simulink model "distributed_project_triangle_adjusted"  (R2025b)
settings: Solver=VariableStepAuto  StartTime=0.0  StopTime=10  RelTol=1e-3  AbsTol=1e-3  EnableMultiTasking=on
model workspace (MAT data in the model file):
  t_now = 10
  v = 1
values from neighbouring files (symbols this model uses):
  m = 20    [FirstRegression.m]
  msg_init =     [distributed_project_adjusted.mat]
  N = min([length(e1), length(e2), length(e3), N_max])    [10_runs_result_for_odometer.m]    (also in cc.m = min(length(e1), length(e2)); distributed_project_adjusted.mat = 100; distributed_stats.m = min([length(e1),length(e2),length(e3)]); ten_runs_result_for_odometer.m)
  r = 0.05    [distributed_project.mat]    (also in distributed_project_adjusted.mat)
undefined symbols (not defined in the file or in its folder): fractalcoef, X, Y, Z
libraries: nesl_utility x52, sm_lib x38, simulink x15, matrix_library x15, mspfiltlib x3, sensorgpslib x3, mspsensorlib x3
(part 3 of 4)

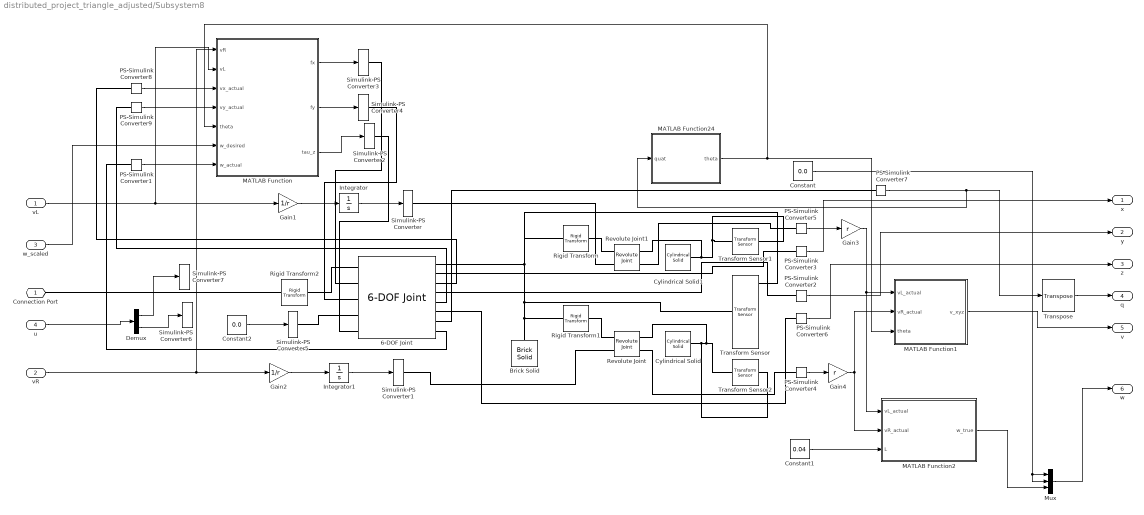
== system distributed_project_triangle_adjusted/Subsystem8 ==
  vL : Inport  PortDimensions=1  SampleTime=0.01
  vR : Inport  Port=2  PortDimensions=1  SampleTime=0.01
  w_scaled : Inport  Port=3
  u : Inport  Port=4  PortDimensions=[2 1]  SampleTime=0.01
  6-DOF Joint : sm_lib/Joints/6-DOF Joint  JointMode=Normal  CompositeWrenchDir=FollowerOnBase  CompositeWrenchFrame=BaseFrame  SenseConstraintForce=off  SenseConstraintTorque=off  SenseTotalForce=off  SenseTotalTorque=off  PxPositionTargetSpecify=on  PxPositionTargetPriority=High  PxPositionTargetValue=0  PxPositionTargetValueUnits=m  PxVelocityTargetSpecify=off  PxVelocityTargetPriority=High  PxVelocityTargetValue=0  PxVelocityTargetValueUnits=m/s  PxEquilibriumPosition=0  PxEquilibriumPositionUnits=m  PxSpringStiffness=0  PxSpringStiffnessUnits=N/m  PxDampingCoefficient=0  PxDampingCoefficientUnits=N/(m/s)  PxLowerLimitSpecify=off  PxLowerLimitBound=-1  PxLowerLimitBoundUnits=m  PxLowerLimitStiffness=1e6  PxLowerLimitStiffnessUnits=N/m  PxLowerLimitDamping=1e3  PxLowerLimitDampingUnits=N/(m/s)  PxLowerLimitTransitionRegionWidth=1e-4  PxLowerLimitTransitionRegionWidthUnits=m  PxUpperLimitSpecify=off  PxUpperLimitBound=1  PxUpperLimitBoundUnits=m  PxUpperLimitStiffness=1e6  PxUpperLimitStiffnessUnits=N/m  PxUpperLimitDamping=1e3  PxUpperLimitDampingUnits=N/(m/s)  PxUpperLimitTransitionRegionWidth=1e-4  PxUpperLimitTransitionRegionWidthUnits=m  PxTorqueActuationMode=InputTorque  PxMotionActuationMode=ComputedMotion  PxSensePosition=on  PxSenseVelocity=on  PxSenseAcceleration=off  PxSenseTorqueForce=off  PxSenseLowerLimitTorqueForce=off  PxSenseUpperLimitTorqueForce=off  PyPositionTargetSpecify=on  PyPositionTargetPriority=High  PyPositionTargetValue=0  PyPositionTargetValueUnits=m  PyVelocityTargetSpecify=off  PyVelocityTargetPriority=High  PyVelocityTargetValue=0  PyVelocityTargetValueUnits=m/s  PyEquilibriumPosition=0  PyEquilibriumPositionUnits=m  PySpringStiffness=0  PySpringStiffnessUnits=N/m  PyDampingCoefficient=0  PyDampingCoefficientUnits=N/(m/s)  PyLowerLimitSpecify=off  PyLowerLimitBound=-1  PyLowerLimitBoundUnits=m  PyLowerLimitStiffness=1e6  PyLowerLimitStiffnessUnits=N/m  PyLowerLimitDamping=1e3  PyLowerLimitDampingUnits=N/(m/s)  PyLowerLimitTransitionRegionWidth=1e-4  PyLowerLimitTransitionRegionWidthUnits=m  PyUpperLimitSpecify=off  PyUpperLimitBound=1  PyUpperLimitBoundUnits=m  PyUpperLimitStiffness=1e6  PyUpperLimitStiffnessUnits=N/m  PyUpperLimitDamping=1e3  PyUpperLimitDampingUnits=N/(m/s)  PyUpperLimitTransitionRegionWidth=1e-4  PyUpperLimitTransitionRegionWidthUnits=m  PyTorqueActuationMode=InputTorque  PyMotionActuationMode=ComputedMotion  PySensePosition=on  PySenseVelocity=on  PySenseAcceleration=off  PySenseTorqueForce=off  PySenseLowerLimitTorqueForce=off  PySenseUpperLimitTorqueForce=off  PzPositionTargetSpecify=on  PzPositionTargetPriority=High  PzPositionTargetValue=0.075  PzPositionTargetValueUnits=m  PzVelocityTargetSpecify=on  PzVelocityTargetPriority=High  PzVelocityTargetValue=0  PzVelocityTargetValueUnits=m/s  PzEquilibriumPosition=0  PzEquilibriumPositionUnits=m  PzSpringStiffness=0  PzSpringStiffnessUnits=N/m  PzDampingCoefficient=0  PzDampingCoefficientUnits=N/(m/s)  PzLowerLimitSpecify=off  PzLowerLimitBound=-1  PzLowerLimitBoundUnits=m  PzLowerLimitStiffness=1e6  PzLowerLimitStiffnessUnits=N/m  PzLowerLimitDamping=1e3  PzLowerLimitDampingUnits=N/(m/s)  PzLowerLimitTransitionRegionWidth=1e-4  PzLowerLimitTransitionRegionWidthUnits=m  PzUpperLimitSpecify=off  PzUpperLimitBound=1  PzUpperLimitBoundUnits=m  PzUpperLimitStiffness=1e6  PzUpperLimitStiffnessUnits=N/m  PzUpperLimitDamping=1e3  PzUpperLimitDampingUnits=N/(m/s)  PzUpperLimitTransitionRegionWidth=1e-4  PzUpperLimitTransitionRegionWidthUnits=m  PzTorqueActuationMode=ComputedTorque  PzMotionActuationMode=InputMotion  PzSensePosition=on  PzSenseVelocity=off  PzSenseAcceleration=off  PzSenseTorqueForce=off  PzSenseLowerLimitTorqueForce=off  PzSenseUpperLimitTorqueForce=off  SphPositionTargetSpecify=on  SphPositionTargetPriority=High  SphPositionTargetRotationMethod=StandardAxis  SphPositionTargetFollAlignAxisA=+X  SphPositionTargetBaseAlignAxisA=+Y  SphPositionTargetFollAlignAxisB=+Y  SphPositionTargetBaseAlignAxisB=+Z  SphPositionTargetRotationStandardAxis=+Z  SphPositionTargetRotationAngle=0.0  SphPositionTargetRotationAngleUnits=rad  SphPositionTargetRotationArbitraryAxis=[0 0 1]  SphPositionTargetRotationSequenceAxes=FollowerAxes  SphPositionTargetRotationSequence=XYX  SphPositionTargetRotationSequenceAngles=[0 0 0]  SphPositionTargetRotationSequenceAnglesUnits=deg  SphPositionTargetRotationMatrix=[1 0 0;0 1 0;0 0 1]  SphPositionTargetQuaternion=[1 0 0 0]  SphVelocityTargetSpecify=off  SphVelocityTargetPriority=High  SphVelocityTargetValue=[0 0 0]  SphVelocityTargetValueUnits=rad/s  SphVelocityTargetInFollowerFrame=on  SphEqPosRotationMethod=None  SphEqPosFollAlignAxisA=+X  SphEqPosBaseAlignAxisA=+Y  SphEqPosFollAlignAxisB=+Y  SphEqPosBaseAlignAxisB=+Z  SphEqPosRotationStandardAxis=+Z  SphEqPosRotationAngle=0  SphEqPosRotationAngleUnits=deg  SphEqPosRotationArbitraryAxis=[0 0 1]  SphEqPosRotationSequenceAxes=FollowerAxes  SphEqPosRotationSequence=XYX  SphEqPosRotationSequenceAngles=[0 0 0]  SphEqPosRotationSequenceAnglesUnits=deg  SphEqPosRotationMatrix=[1 0 0;0 1 0;0 0 1]  SphEqPosQuaternion=[1 0 0 0]  SphSpringStiffness=0  SphSpringStiffnessUnits=N*m/deg  SphDampingCoefficient=0  SphDampingCoefficientUnits=N*m/(deg/s)  SphLowerLimitSpecify=off  SphLowerLimitBound=15  SphLowerLimitBoundUnits=deg  SphLowerLimitStiffness=1e4  SphLowerLimitStiffnessUnits=N*m/deg  SphLowerLimitDamping=10  SphLowerLimitDampingUnits=N*m/(deg/s)  SphLowerLimitTransitionRegionWidth=0.1  SphLowerLimitTransitionRegionWidthUnits=deg  SphUpperLimitSpecify=off  SphUpperLimitBound=45  SphUpperLimitBoundUnits=deg  SphUpperLimitStiffness=1e4  SphUpperLimitStiffnessUnits=N*m/deg  SphUpperLimitDamping=10  SphUpperLimitDampingUnits=N*m/(deg/s)  SphUpperLimitTransitionRegionWidth=0.1  SphUpperLimitTransitionRegionWidthUnits=deg  SphTorqueActuationMode=InputTorque  SphActuateTorqueX=off  SphActuateTorqueY=off  SphActuateTorqueZ=on  SphActuateTorque=off  SphActuationFrame=BaseFrame  SphSensePosition=on  SphSenseVelocityX=off  SphSenseVelocityY=off  SphSenseVelocityZ=on  SphSenseVelocity=off  SphSenseAccelerationX=off  SphSenseAccelerationY=off  SphSenseAccelerationZ=off  SphSenseAcceleration=off  SphSenseLowerLimitTorqueMag=off  SphSenseUpperLimitTorqueMag=off  SphSensingFrame=BaseFrame
  Brick Solid : sm_lib/Body Elements/Brick Solid  BrickDimensions=[0.3 0.15 0.2]  BrickDimensionsUnits=m  ExportEntireGeometry=off  InertiaType=CalculateFromGeometry  BasedOnType=Density  Density=1000  DensityUnits=kg/m^3  Mass=1  MassUnits=kg  CenterOfMass=[0 0 0]  CenterOfMassUnits=m  MomentsOfInertia=[1 1 1]  MomentsOfInertiaUnits=kg*m^2  ProductsOfInertia=[0 0 0]  ProductsOfInertiaUnits=kg*m^2  GraphicType=FromGeometry  MarkerShape=Sphere  MarkerSize=10  GraphicVisPropType=AdvancedVisualProperties  GraphicDiffuseColor=[0.5 0.5 0.5]  GraphicOpacity=1.0  GraphicSpecularColor=[0.5 0.5 0.5 1.0]  GraphicAmbientColor=[0.15 0.15 0.15 1.0]  GraphicEmissiveColor=[0.0 0.0 0.0 1.0]  GraphicShininess=75  DoExposeReferenceFrame=on  SerializedFrames=<Frames/>
  Constant : Constant  Value=0.0  SampleTime=0.01
  Constant1 : Constant  Value=0.04  SampleTime=0.01
  Constant2 : Constant  Value=0.0  SampleTime=0.01
  Cylindrical Solid : sm_lib/Body Elements/Cylindrical Solid  CylinderRadius=0.05  CylinderRadiusUnits=m  CylinderLength=0.04  CylinderLengthUnits=m  ExportEntireGeometry=off  InertiaType=CalculateFromGeometry  BasedOnType=Density  Density=1000  DensityUnits=kg/m^3  Mass=1  MassUnits=kg  CenterOfMass=[0 0 0]  CenterOfMassUnits=m  MomentsOfInertia=[1 1 1]  MomentsOfInertiaUnits=kg*m^2  ProductsOfInertia=[0 0 0]  ProductsOfInertiaUnits=kg*m^2  GraphicType=FromGeometry  MarkerShape=Sphere  MarkerSize=10  GraphicVisPropType=SimpleVisualProperties  GraphicDiffuseColor=[0.5 0.5 0.5]  GraphicOpacity=1  GraphicSpecularColor=[0.5 0.5 0.5 1.0]  GraphicAmbientColor=[0.15 0.15 0.15 1.0]  GraphicEmissiveColor=[0.0 0.0 0.0 1.0]  GraphicShininess=75  DoExposeReferenceFrame=on  SerializedFrames=<Frames/>
  Cylindrical Solid1 : sm_lib/Body Elements/Cylindrical Solid  CylinderRadius=0.05  CylinderRadiusUnits=m  CylinderLength=0.04  CylinderLengthUnits=m  ExportEntireGeometry=off  InertiaType=CalculateFromGeometry  BasedOnType=Density  Density=1000  DensityUnits=kg/m^3  Mass=1  MassUnits=kg  CenterOfMass=[0 0 0]  CenterOfMassUnits=m  MomentsOfInertia=[1 1 1]  MomentsOfInertiaUnits=kg*m^2  ProductsOfInertia=[0 0 0]  ProductsOfInertiaUnits=kg*m^2  GraphicType=FromGeometry  MarkerShape=Sphere  MarkerSize=10  GraphicVisPropType=SimpleVisualProperties  GraphicDiffuseColor=[0.5 0.5 0.5]  GraphicOpacity=1  GraphicSpecularColor=[0.5 0.5 0.5 1.0]  GraphicAmbientColor=[0.15 0.15 0.15 1.0]  GraphicEmissiveColor=[0.0 0.0 0.0 1.0]  GraphicShininess=75  DoExposeReferenceFrame=on  SerializedFrames=<Frames/>
  Demux : Demux  Outputs=2
  Gain1 : Gain  Gain=1/r
  Gain2 : Gain  Gain=1/r
  Gain3 : Gain  Gain=r
  Gain4 : Gain  Gain=r
  Integrator : Integrator
  Integrator1 : Integrator
  MATLAB Function : MATLAB Function  TreatAsAtomicUnit=on
  MATLAB Function1 : MATLAB Function  TreatAsAtomicUnit=on
  MATLAB Function2 : MATLAB Function  TreatAsAtomicUnit=on
  MATLAB Function24 : MATLAB Function  TreatAsAtomicUnit=on
  Mux : Mux  Inputs=3
  PS-Simulink Converter{1..9} (9 alike) : nesl_utility/PS-Simulink Converter  PhysicalDomain=network_engine_domain  SubClassName=ps_output  LeftPortType=input  RightPortType=output  PseudoPeriodic=off  Frequencies=[]  VectorFormat=inherit  Unit=inherit  AffineConversion=off
  Revolute Joint : sm_lib/Joints/Revolute Joint  JointMode=Normal  CompositeWrenchDir=FollowerOnBase  CompositeWrenchFrame=BaseFrame  SenseConstraintForce=off  SenseConstraintTorque=off  SenseTotalForce=off  SenseTotalTorque=off  PositionTargetSpecify=off  PositionTargetPriority=High  PositionTargetValue=0  PositionTargetValueUnits=rad  VelocityTargetSpecify=off  VelocityTargetPriority=High  VelocityTargetValue=0  VelocityTargetValueUnits=rad/s  EquilibriumPosition=0  EquilibriumPositionUnits=deg  SpringStiffness=0  SpringStiffnessUnits=N*m/deg  DampingCoefficient=0  DampingCoefficientUnits=N*m/(deg/s)  LowerLimitSpecify=off  LowerLimitBound=-90  LowerLimitBoundUnits=deg  LowerLimitStiffness=1e4  LowerLimitStiffnessUnits=N*m/deg  LowerLimitDamping=10  LowerLimitDampingUnits=N*m/(deg/s)  LowerLimitTransitionRegionWidth=0.1  LowerLimitTransitionRegionWidthUnits=deg  UpperLimitSpecify=off  UpperLimitBound=90  UpperLimitBoundUnits=deg  UpperLimitStiffness=1e4  UpperLimitStiffnessUnits=N*m/deg  UpperLimitDamping=10  UpperLimitDampingUnits=N*m/(deg/s)  UpperLimitTransitionRegionWidth=0.1  UpperLimitTransitionRegionWidthUnits=deg  TorqueActuationMode=ComputedTorque  MotionActuationMode=InputMotion  SensePosition=off  SenseVelocity=on  SenseAcceleration=off  SenseTorqueForce=off  SenseLowerLimitTorqueForce=off  SenseUpperLimitTorqueForce=off
  Revolute Joint1 : sm_lib/Joints/Revolute Joint  JointMode=Normal  CompositeWrenchDir=FollowerOnBase  CompositeWrenchFrame=BaseFrame  SenseConstraintForce=off  SenseConstraintTorque=off  SenseTotalForce=off  SenseTotalTorque=off  PositionTargetSpecify=off  PositionTargetPriority=High  PositionTargetValue=0  PositionTargetValueUnits=rad  VelocityTargetSpecify=off  VelocityTargetPriority=High  VelocityTargetValue=0  VelocityTargetValueUnits=rad/s  EquilibriumPosition=0  EquilibriumPositionUnits=deg  SpringStiffness=0  SpringStiffnessUnits=N*m/deg  DampingCoefficient=0  DampingCoefficientUnits=N*m/(deg/s)  LowerLimitSpecify=off  LowerLimitBound=-90  LowerLimitBoundUnits=deg  LowerLimitStiffness=1e4  LowerLimitStiffnessUnits=N*m/deg  LowerLimitDamping=10  LowerLimitDampingUnits=N*m/(deg/s)  LowerLimitTransitionRegionWidth=0.1  LowerLimitTransitionRegionWidthUnits=deg  UpperLimitSpecify=off  UpperLimitBound=90  UpperLimitBoundUnits=deg  UpperLimitStiffness=1e4  UpperLimitStiffnessUnits=N*m/deg  UpperLimitDamping=10  UpperLimitDampingUnits=N*m/(deg/s)  UpperLimitTransitionRegionWidth=0.1  UpperLimitTransitionRegionWidthUnits=deg  TorqueActuationMode=ComputedTorque  MotionActuationMode=InputMotion  SensePosition=off  SenseVelocity=on  SenseAcceleration=off  SenseTorqueForce=off  SenseLowerLimitTorqueForce=off  SenseUpperLimitTorqueForce=off
  Rigid Transform : sm_lib/Frames and Transforms/Rigid Transform  RotationMethod=RotationSequence  FollAlignAxisA=+X  BaseAlignAxisA=+Y  FollAlignAxisB=+Y  BaseAlignAxisB=+Z  RotationStandardAxis=+Z  RotationAngle=0  RotationAngleUnits=deg  RotationArbitraryAxis=[0 0 1]  RotationSequenceAxes=FollowerAxes  RotationSequence=XZY  RotationSequenceAngles=[90 90 0]  RotationSequenceAnglesUnits=deg  RotationMatrix=[1 0 0;0 1 0;0 0 1]  Quaternion=[1 0 0 0]  TranslationMethod=Cartesian  TranslationCartesianOffset=[0 0.095 0]  TranslationCartesianOffsetUnits=m  TranslationStandardAxis=+Z  TranslationStandardOffset=0  TranslationStandardOffsetUnits=m  TranslationROffset=0  TranslationROffsetUnits=m  TranslationThetaOffset=0  TranslationThetaOffsetUnits=deg  TranslationZOffset=0  TranslationZOffsetUnits=m
  Rigid Transform1 : sm_lib/Frames and Transforms/Rigid Transform  RotationMethod=RotationSequence  FollAlignAxisA=+X  BaseAlignAxisA=+Y  FollAlignAxisB=+Y  BaseAlignAxisB=+Z  RotationStandardAxis=+Z  RotationAngle=0  RotationAngleUnits=deg  RotationArbitraryAxis=[0 0 1]  RotationSequenceAxes=FollowerAxes  RotationSequence=XZY  RotationSequenceAngles=[90 90 0]  RotationSequenceAnglesUnits=deg  RotationMatrix=[1 0 0;0 1 0;0 0 1]  Quaternion=[1 0 0 0]  TranslationMethod=Cartesian  TranslationCartesianOffset=[0 -0.095 0]  TranslationCartesianOffsetUnits=m  TranslationStandardAxis=+Z  TranslationStandardOffset=0  TranslationStandardOffsetUnits=m  TranslationROffset=0  TranslationROffsetUnits=m  TranslationThetaOffset=0  TranslationThetaOffsetUnits=deg  TranslationZOffset=0  TranslationZOffsetUnits=m
  Rigid Transform2 : sm_lib/Frames and Transforms/Rigid Transform  RotationMethod=None  FollAlignAxisA=+X  BaseAlignAxisA=+Y  FollAlignAxisB=+Y  BaseAlignAxisB=+Z  RotationStandardAxis=+Z  RotationAngle=0  RotationAngleUnits=deg  RotationArbitraryAxis=[0 0 1]  RotationSequenceAxes=FollowerAxes  RotationSequence=XZY  RotationSequenceAngles=[90 0 0]  RotationSequenceAnglesUnits=deg  RotationMatrix=[1 0 0;0 1 0;0 0 1]  Quaternion=[1 0 0 0]  TranslationMethod=None  TranslationCartesianOffset=[0 0 0]  TranslationCartesianOffsetUnits=m  TranslationStandardAxis=+Z  TranslationStandardOffset=0.075  TranslationStandardOffsetUnits=m  TranslationROffset=0  TranslationROffsetUnits=m  TranslationThetaOffset=0  TranslationThetaOffsetUnits=deg  TranslationZOffset=0  TranslationZOffsetUnits=m
  Simulink-PS Converter{,1..7} (8 alike) : nesl_utility/Simulink-PS Converter  PhysicalDomain=network_engine_domain  SubClassName=ps_input  LeftPortType=input  RightPortType=output  PseudoPeriodic=off  Frequencies=[]  NoiseDistribution=none  NoiseParameters=[]  Unit=1  AffineConversion=on  FilteringAndDerivatives=filter  SimscapeFilterOrder=2  InputFilterTimeConstant=0.001  UdotUserProvided=0
  Transform Sensor : sm_lib/Frames and Transforms/Transform Sensor  MeasurementFrame=World  RotationSequence=XZY  SenseAngle=off  SenseAxis=off  SenseQ=off  SenseR=off  SenseRotationSequence=off  SenseOmegaX=off  SenseOmegaY=off  SenseOmegaZ=off  SenseOmega=off  SenseQDot=off  SenseRDot=off  SenseRotationSequenceDot=off  SenseAlphaX=off  SenseAlphaY=off  SenseAlphaZ=off  SenseAlpha=off  SenseQDDot=off  SenseRDDot=off  SenseX=on  SenseY=on  SenseZ=on  SenseXYZ=off  SenseRad=off  SenseAzim=off  SenseDist=off  SenseInc=off  SenseXDot=off  SenseYDot=off  SenseZDot=off  SenseXYZDot=off  SenseRadDot=off  SenseAzimDot=off  SenseDistDot=off  SenseIncDot=off  SenseXDDot=off  SenseYDDot=off  SenseZDDot=off  SenseXYZDDot=off  SenseRadDDot=off  SenseAzimDDot=off  SenseDistDDot=off  SenseIncDDot=off
  Transform Sensor1 : sm_lib/Frames and Transforms/Transform Sensor  MeasurementFrame=World  RotationSequence=XZY  SenseAngle=off  SenseAxis=off  SenseQ=off  SenseR=off  SenseRotationSequence=off  SenseOmegaX=off  SenseOmegaY=off  SenseOmegaZ=off  SenseOmega=off  SenseQDot=off  SenseRDot=off  SenseRotationSequenceDot=off  SenseAlphaX=off  SenseAlphaY=off  SenseAlphaZ=off  SenseAlpha=off  SenseQDDot=off  SenseRDDot=off  SenseX=off  SenseY=off  SenseZ=off  SenseXYZ=off  SenseRad=off  SenseAzim=off  SenseDist=off  SenseInc=off  SenseXDot=off  SenseYDot=off  SenseZDot=off  SenseXYZDot=off  SenseRadDot=off  SenseAzimDot=off  SenseDistDot=off  SenseIncDot=off  SenseXDDot=off  SenseYDDot=off  SenseZDDot=off  SenseXYZDDot=off  SenseRadDDot=off  SenseAzimDDot=off  SenseDistDDot=off  SenseIncDDot=off
  Transform Sensor2 : sm_lib/Frames and Transforms/Transform Sensor  MeasurementFrame=World  RotationSequence=XZY  SenseAngle=off  SenseAxis=off  SenseQ=off  SenseR=off  SenseRotationSequence=off  SenseOmegaX=off  SenseOmegaY=off  SenseOmegaZ=off  SenseOmega=off  SenseQDot=off  SenseRDot=off  SenseRotationSequenceDot=off  SenseAlphaX=off  SenseAlphaY=off  SenseAlphaZ=off  SenseAlpha=off  SenseQDDot=off  SenseRDDot=off  SenseX=off  SenseY=off  SenseZ=off  SenseXYZ=off  SenseRad=off  SenseAzim=off  SenseDist=off  SenseInc=off  SenseXDot=off  SenseYDot=off  SenseZDot=off  SenseXYZDot=off  SenseRadDot=off  SenseAzimDot=off  SenseDistDot=off  SenseIncDot=off  SenseXDDot=off  SenseYDDot=off  SenseZDDot=off  SenseXYZDDot=off  SenseRadDDot=off  SenseAzimDDot=off  SenseDistDDot=off  SenseIncDDot=off
  Transpose : matrix_library/Transpose
  Connection Port : PMIOPort  Side=Left
  x : Outport
  y : Outport  Port=2
  z : Outport  Port=3
  q : Outport  Port=4  PortDimensions=[1 4]
  v : Outport  Port=5  PortDimensions=[3 1]
  w : Outport  Port=6  PortDimensions=[3 1]
  wires:
  PS-Simulink Converter3/1 -> x/1
  PS-Simulink Converter2/1 -> y/1
  Constant/1 -> Mux/2, Mux/1
  vL/1 -> Gain1/1, MATLAB Function/2(vL)
  vR/1 -> MATLAB Function/1(vR), Gain2/1
  Gain1/1 -> Integrator/1
  Gain2/1 -> Integrator1/1
  Integrator/1 -> Simulink-PS Converter/1
  Integrator1/1 -> Simulink-PS Converter1/1
  PS-Simulink Converter5/1 -> Gain3/1
  PS-Simulink Converter4/1 -> Gain4/1
  Gain3/1 -> MATLAB Function2/1(vL_actual), MATLAB Function1/1(vL_actual)
  MATLAB Function1/1(v_xyz) -> v/1
  Gain4/1 -> MATLAB Function2/2(vR_actual), MATLAB Function1/2(vR_actual)
  Constant1/1 -> MATLAB Function2/3(L)
  MATLAB Function2/1(w_true) -> Mux/3
  Mux/1 -> w/1
  PS-Simulink Converter7/1 -> MATLAB Function24/1(quat), Transpose/1
  Transpose/1 -> q/1
  MATLAB Function/3(tau_z) -> Simulink-PS Converter2/1
  MATLAB Function24/1(theta) -> MATLAB Function/5(theta), MATLAB Function1/3(theta)
  PS-Simulink Converter8/1 -> MATLAB Function/3(vx_actual)
  PS-Simulink Converter9/1 -> MATLAB Function/4(vy_actual)
  w_scaled/1 -> MATLAB Function/6(w_desired)
  MATLAB Function/1(fx) -> Simulink-PS Converter3/1
  MATLAB Function/2(fy) -> Simulink-PS Converter4/1
  PS-Simulink Converter6/1 -> z/1
  PS-Simulink Converter1/1 -> MATLAB Function/7(w_actual)
  Constant2/1 -> Simulink-PS Converter5/1
  u/1 -> Demux/1
  Demux/1 -> Simulink-PS Converter7/1
  Demux/2 -> Simulink-PS Converter6/1
  connections:
  Cylindrical Solid/RConn1 -- Transform Sensor2/RConn1 -- Revolute Joint/RConn1 -- Transform Sensor2/LConn1
  Transform Sensor1/LConn1 -- Cylindrical Solid1/RConn1 -- Revolute Joint1/RConn1 -- Transform Sensor1/RConn1
  Rigid Transform/RConn1 -- Revolute Joint1/LConn1
  Revolute Joint/LConn1 -- Rigid Transform1/RConn1
  Transform Sensor/LConn1 -- Rigid Transform/LConn1 -- Transform Sensor/RConn1 -- 6-DOF Joint/RConn1 -- Brick Solid/RConn1 -- Rigid Transform1/LConn1
  Rigid Transform2/LConn1 -- Connection Port/RConn1
  Revolute Joint/RConn2 -- PS-Simulink Converter4/LConn1
  Revolute Joint1/RConn2 -- PS-Simulink Converter5/LConn1
  6-DOF Joint/RConn7 -- PS-Simulink Converter7/LConn1
  PS-Simulink Converter1/LConn1 -- 6-DOF Joint/RConn8
  6-DOF Joint/RConn3 -- PS-Simulink Converter8/LConn1
  6-DOF Joint/RConn5 -- PS-Simulink Converter9/LConn1
  Revolute Joint1/LConn2 -- Simulink-PS Converter/RConn1
  Revolute Joint/LConn2 -- Simulink-PS Converter1/RConn1
  6-DOF Joint/RConn2 -- PS-Simulink Converter3/LConn1
  6-DOF Joint/RConn4 -- PS-Simulink Converter2/LConn1
  6-DOF Joint/RConn6 -- PS-Simulink Converter6/LConn1
  6-DOF Joint/LConn1 -- Rigid Transform2/RConn1
  Simulink-PS Converter5/RConn1 -- 6-DOF Joint/LConn4
  Simulink-PS Converter2/RConn1 -- 6-DOF Joint/LConn5
  Simulink-PS Converter3/RConn1 -- 6-DOF Joint/LConn2
  Simulink-PS Converter4/RConn1 -- 6-DOF Joint/LConn3

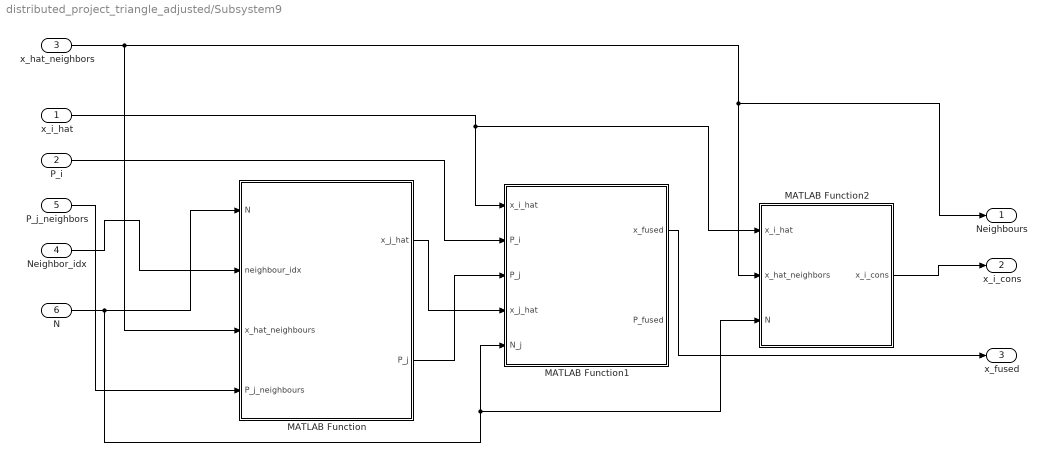
== system distributed_project_triangle_adjusted/Subsystem9 ==
  x_i_hat : Inport
  P_i : Inport  Port=2
  x_hat_neighbors : Inport  Port=3
  Neighbor_idx : Inport  Port=4
  P_j_neighbors : Inport  Port=5
  N : Inport  Port=6
  MATLAB Function : MATLAB Function  TreatAsAtomicUnit=on
  MATLAB Function1 : MATLAB Function  TreatAsAtomicUnit=on
  MATLAB Function2 : MATLAB Function  TreatAsAtomicUnit=on
  Neighbours : Outport
  x_i_cons : Outport  Port=2
  x_fused : Outport  Port=3
  wires:
  Neighbor_idx/1 -> MATLAB Function/2(neighbour_idx)
  x_i_hat/1 -> MATLAB Function2/1(x_i_hat), MATLAB Function1/1(x_i_hat)
  x_hat_neighbors/1 -> MATLAB Function/3(x_hat_neighbours), Neighbours/1, MATLAB Function2/2(x_hat_neighbors)
  MATLAB Function/1(x_j_hat) -> MATLAB Function1/4(x_j_hat)
  P_j_neighbors/1 -> MATLAB Function/4(P_j_neighbours)
  MATLAB Function1/1(x_fused) -> x_fused/1
  P_i/1 -> MATLAB Function1/2(P_i)
  MATLAB Function/2(P_j) -> MATLAB Function1/3(P_j)
  MATLAB Function2/1(x_i_cons) -> x_i_cons/1
  N/1 -> MATLAB Function2/3(N), MATLAB Function1/5(N_j), MATLAB Function/1(N)

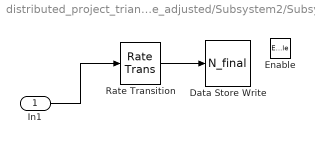
== system distributed_project_triangle_adjusted/Subsystem2/Subsystem ==
  In1 : Inport
  Enable : EnablePort
  Data Store Write : DataStoreWrite  DataStoreName=N_final  SampleTime=0.01  IndexOptions=Index vector (dialog)  Indices=1  OutputSizes=1
  Rate Transition : RateTransition  OutPortSampleTime=0.01
  wires:
  Rate Transition/1 -> Data Store Write/1
  In1/1 -> Rate Transition/1

== matlab function distributed_project_triangle_adjusted/Subsystem7/MATLAB Function2 ==
  data: x_i_hat input; x_i_cons output; x_hat_neighbors input; N input
function x_i_cons  = consensus_update(x_i_hat, x_hat_neighbors,N)
% CONSENSUS_BLOCK - Multi-agent consensus update
%
% Inputs:
%   x_hat_i         - current state estimate of agent i (scalar or vector)
%   x_hat_neighbors - matrix of neighbor estimates (each column = neighbor)
%   a_ij            - vector of weights for each neighbor
%   gain            - epsilon (continuous) or gamma (discrete)
%   dt              - timestep (for discrete integration if mode='continuous')
%   mode            - 'continuous' or 'discrete'
%
% Output:
%   x_hat_next      - updated state estimate of agent i

% Compute weighted difference with neighbors
gamma = 0.05;
N_neighbours = size(x_hat_neighbors, 2); 
a_ij = zeros(1:N_neighbours);
x_i_cons = zeros(size(x_i_hat));
% number of neighbors
a_ij(:) = 1/N_neighbours;  
diff = zeros(size(x_i_hat));
    for j = 1:N-1
        diff = diff + a_ij(j) * (x_hat_neighbors(:,j) - x_i_hat);
            
    end
x_i_cons = x_i_hat + gamma * diff;

end

== matlab function distributed_project_triangle_adjusted/MATLAB Function3 ==
  data: x_i_cons input; x_hat_neighbors input; N_all input; x_c output
function x_c = centroid_estimator(x_i_cons, x_hat_neighbors, N_all)
%#codegen
%% Inputs:
%%   x_i_cons        - own consensus state  (5×1)
%%   x_hat_neighbors - neighbour states     (5×N_neighbors)
%%                     columns 1..N_neighbors are valid
%%   N_neighbors     - actual neighbour count (not N_max)
%%
%% Output:
%%   x_c             - centroid (2×1)

%% Own position — always (2×1) after explicit indexing
own_pos = [x_i_cons(1); x_i_cons(2)];   % explicit 2×1, no reshape


%% Sum own position
pos_sum = own_pos;

%% Add each neighbour position explicitly
for j = 1:N_all-1
    pos_sum = pos_sum + [x_hat_neighbors(1,j); x_hat_neighbors(2,j)];
end

%% Average over total count
x_c   = pos_sum / N_all;
end

== matlab function distributed_project_triangle_adjusted/MATLAB Function1 ==
  data: x output; lat input; y output; lon input
function [x,y] = getXY(lat, lon)

% Reference point
persistent lat0 lon0 initialized

if isempty(initialized)
    lat0 = lat;
    lon0 = lon;
    initialized = true;
end



% Convert to radians
lat0_rad = deg2rad(lat0);
lon0_rad = deg2rad(lon0);
lat_rad  = deg2rad(lat);
lon_rad  = deg2rad(lon);

% Earth radius
R = 6371000; % meters

% Compute local x, y
lat_avg = (lat_rad + lat0_rad)/2;
x = R * (lon_rad - lon0_rad) * cos(lat_avg); % east
y = R * (lat_rad - lat0_rad);                 % north

== matlab function distributed_project_triangle_adjusted/MATLAB Function2 ==
  data: msg_in input; x_hat_neighbors output; neighbor_idx output; P_j_neighbours output; N output; my_id input; t_now input size=1
function [x_hat_neighbors, neighbor_idx, P_j_neighbours, N] = ...
         receive_msg(msg_in, my_id, t_now)
%#codegen

%% Fixed dimensions — must be constants for codegen
MAX_AGENTS  = 7;
STATE_DIM   = 3;
P_DIM       = 3;
T_WINDOW    = 5.0;   % seconds — max message age

N = 0;

for i = 1:length(msg_in)
    if msg_in(i).ID ~= 0   % assume ID=0 means empty slot
        N = N + 1;
    end
end


%% Fixed-size outputs — codegen requires known dimensions
x_hat_neighbors = zeros(STATE_DIM, MAX_AGENTS);
P_j_neighbours  = zeros(P_DIM, P_DIM, MAX_AGENTS);
neighbor_idx    = zeros(1, MAX_AGENTS);
N_neighbors     = 0;




%% Persistent store — holds latest message per agent slot
%% Indexed by agent ID (1..MAX_AGENTS)
persistent latest_x latest_P latest_t latest_valid

if isempty(latest_x)
    latest_x     = zeros(STATE_DIM, MAX_AGENTS);
    latest_P     = zeros(P_DIM, P_DIM, MAX_AGENTS);
    latest_t     = -inf(1, MAX_AGENTS);   % never received
    latest_valid = zeros(1, MAX_AGENTS);  % 0 = no data
end

%% ── Step 1: Update persistent store with incoming messages ────────
for k = 1:length(msg_in)
    id = msg_in(k).ID;

    %% Skip invalid IDs
    if id < 1 || id > N
        continue;
    end

    %% Skip own messages
    if id == my_id
        continue;
    end

    %% Keep only the latest message per ID
    if msg_in(k).t > latest_t(id)
        latest_x(:, id)      = msg_in(k).x;
        latest_P(:, :, id)   = msg_in(k).P;
        latest_t(id)         = msg_in(k).t;
        latest_valid(id)     = 1;
    end
end

%% ── Step 2: Collect valid neighbours within time window ───────────
for id = 1:N

    %% Skip self
    if id == my_id
        continue;
    end

    %% Skip slots never received
    if latest_valid(id) == 0
        continue;
    end

    %% Skip stale messages
    msg_age = t_now - latest_t(id);
    if msg_age > T_WINDOW || msg_age < 0
        continue;
    end

    %% Valid neighbour — add to output
    N_neighbors = N_neighbors + 1;
    x_hat_neighbors(:, N_neighbors) = latest_x(:, id);
    P_j_neighbours(:,:, N_neighbors) = latest_P(:,:, id);
    neighbor_idx(N_neighbors) = id;
end





end

== matlab function distributed_project_triangle_adjusted/Subsystem2/MATLAB Function8 ==
  data: N_i input; N_final output; trigger output
function [N_final, trigger] = convergence_detector(N_i)

%#codegen

% PARAMETERS
k = 5;   % number of steps for stability

% PERSISTENT MEMORY
persistent buffer count

    if isempty(buffer)
        buffer = zeros(k,1);
        count = 0;
    end

% SHIFT BUFFER (like Unit Delay chain)
buffer = [buffer(2:end); N_i];

% CHECK IF ALL VALUES SAME


    if all(buffer == buffer(1))
        count = count + 1;
    else
        count = 0;
    end

    % TRIGGER WHEN STABLE
    if count >= 1   % already stable for k steps
        trigger = 1;
        N_final = buffer(end);
    else
        trigger = 0;
        N_final = N_i;
    end

end

== matlab function distributed_project_triangle_adjusted/MATLAB Function4 ==
  data: ID_i input; delta_i output double; N input; formation input
function delta_i = formation_calculator(ID_i, N, formation)
    %#codegen
    
    delta_i = [0; 0];
    
    if N <= 0 || ID_i < 1 || ID_i > N || N == 1
        return;
    end
    spacing = 0.5;
    switch formation
        case 1  % LINE (N ≤ 2)
            center = (N - 1) / 2;
            delta_i = double([(ID_i - 1 - center) * spacing; 0]);
            
        case 2  % CIRCLE (N ≥ 5)
            radius = spacing * N / (2 * pi);
            theta = 2 * pi * (ID_i - 1) / N;
            delta_i = radius * [cos(double(theta)); sin(double(theta))];
            
        case 3  % SQUARE (N = 4)
            half = spacing / 2;
            corners = [ half, -half, -half,  half;   % x-coordinates
                       -half, -half,  half,  half];  % y-coordinates
            delta_i = corners(:, ID_i);
            
        case 4  % TRIANGLE (N = 3)
            side = spacing * 2;
            h = sqrt(3) / 2 * side;
            vertices = [0,   -side/2,  side/2;    % x-coordinates
                       2*h/3, -h/3,   -h/3];     % y-coordinates
            delta_i = vertices(:, ID_i);
            
        otherwise
            delta_i = [0; 0];
    end
end

== matlab function distributed_project_triangle_adjusted/MATLAB Function5 ==
  data: N_final input; formation output
function formation = formation_selector(N_final)


    if N_final <= 0
        formation = 0;  % Invalid
        warning('Invalid number of agents: %d', N_final);
        return;
    end

    if N_final <= 2
        formation = 1;
    elseif N_final == 3
        formation = 4;
    elseif N_final == 4
        formation = 3;
    else
        formation = 2;
    end

end

== matlab function distributed_project_triangle_adjusted/MATLAB Function6 ==
  data: x_fused input; ei_pos_f output size=[2 1]; x_c input; delta_i input; ei_norm output; x_c_raw input
function [ei_pos_f, ei_norm] = formation_error_calculator(...
                               x_fused, x_c, delta_i, x_c_raw)
%#codegen
persistent ei_prev;
if isempty(ei_prev)
    ei_prev = zeros(2,1);
end
ei_pos_raw = (x_c + delta_i) - x_fused(1:2);

%% Low-pass filter — smooth noise
alpha    = 0.167;   % Ts=0.01, tau=0.05s
ei_pos_f = (1-alpha)*ei_prev + alpha*ei_pos_raw;

%% Use raw norm for threshold (not filtered)
ei_norm = norm((x_c_raw + delta_i) - x_fused(1:2));
ei_prev = ei_pos_f;
end

== matlab function distributed_project_triangle_adjusted/MATLAB Function7 ==
  data: ei_pos input; ei_vel input; kp input; kd input; L input; vL output size=1; vR output size=1; theta input; w_scaled output; u output
function [vL, vR, w_scaled, u] = control_law(ei_pos, ei_vel, kp, kd, L, theta)
%#codegen

u = [0.0; 0.0];
w_scaled = double(0);
vL = double(0);
vR = double(0);

%% Deadband for spacing=0.3m
e_dead = 0.08;
if norm(ei_pos) < e_dead
    return;
end

u = kp * ei_pos - kd * ei_vel;

%% Tighter saturation for small formation
u_max  = 0.4;
u_norm = sqrt(u(1)^2 + u(2)^2);
if u_norm > u_max
    u = u * (u_max / u_norm);
end

v_lin =  cos(theta)*u(1) + sin(theta)*u(2);
w     = -sin(theta)*u(1) + cos(theta)*u(2);

w_scaled = w / (L/2);

v_max = 0.4;     % slower for small formation
w_max = 0.4;
v_lin    = max(-v_max, min(v_max, v_lin));
w_scaled = max(-w_max, min(w_max, w_scaled));

vL = v_lin - (L/2)*w_scaled;
vR = v_lin + (L/2)*w_scaled;
end

== matlab function distributed_project_triangle_adjusted/MATLAB Function10 ==
  data: quat input; theta output
function theta = quat_to_angle(quat)
%#codegen

% normalize (important if coming from simulation)
quat = quat / norm(quat);

w = quat(1);
z = quat(4);

theta = 2 * atan2(z, w);

end

== matlab function distributed_project_triangle_adjusted/Subsystem/MATLAB Function1 ==
  data: pos_x input; x_next output; pos_y input; theta input; v input; a input; w input; P_next output; gyro_bias input
function [x_next, P_next] = local_ekf_predict(pos_x,pos_y, theta, v, a, w, gyro_bias)
% MOTION_UPDATE: Predicts the next state and covariance for a 2D vehicle
%
% Inputs:
%   x  - current state [x; y; theta; v]
%   P  - current state covariance (4x4)
%   u  - control input [a; omega] (acceleration, angular rate)
%   Q  - process noise covariance (4x4)
%   dt - time step Δt
%
% Outputs:
%   x_next - predicted next state
%   P_next - predicted next covariance

dt = 0.01;
%% In PreLoadFcn or MATLAB workspace:

sigma_x     = 0.01;
sigma_y     = 0.01;
sigma_theta = 0.005;

Q = diag([sigma_x^2*dt;
            sigma_y^2*dt;
                sigma_theta^2*dt]);
% Make P persistent across calls
persistent P;
    if isempty(P)
        P = eye(3) * 0.1;  % initialize first time
    end

% State prediction (nonlinear)
x_next = zeros(3,1);

              % angular velocity (yaw)
bias_z = gyro_bias(3);      % gyro bias (yaw)
v = norm(v);
a = norm(a);
x_next(1) = pos_x + v * cos(theta) * dt;
x_next(2) = pos_y + v * sin(theta) * dt;
x_next(3) = theta + w * dt;
%x_next(4) = v + a * dt;
%x_next(5) = bias_z;

% Jacobian F_k = ∂f/∂x
A = [ 1, 0, -v*sin(theta)*dt;
      0, 1,  v*cos(theta)*dt;
      0, 0,               1];               


% Covariance prediction
P_next = A * P * A' + Q;
P = P_next;
end

== matlab function distributed_project_triangle_adjusted/MATLAB Function12 ==
  data: x_c_raw input; x_c_out output size=[2, 1]; all_converged input; x_c_raw output
function [x_c_out, x_c_raw] = centroid_manager(x_c_raw, all_converged)
%#codegen

persistent x_c_latched is_latched;
if isempty(x_c_latched)
    x_c_latched = zeros(2,1);
    is_latched  = false;
end

if all_converged && ~is_latched
    %% Latch centroid at moment of convergence
    x_c_latched = x_c_raw;
    is_latched  = true;
end

if is_latched
    x_c_out = x_c_latched;
else
    x_c_out = x_c_raw;
end
end

== matlab function distributed_project_triangle_adjusted/MATLAB Function13 ==
  data: x_i_cons input; x_hat_neighbors input; N_all input; x_c output
function x_c = centroid_estimator(x_i_cons, x_hat_neighbors, N_all)
%#codegen
%% Inputs:
%%   x_i_cons        - own consensus state  (5×1)
%%   x_hat_neighbors - neighbour states     (5×N_neighbors)
%%                     columns 1..N_neighbors are valid
%%   N_neighbors     - actual neighbour count (not N_max)
%%
%% Output:
%%   x_c             - centroid (2×1)

%% Own position — always (2×1) after explicit indexing
own_pos = [x_i_cons(1); x_i_cons(2)];   % explicit 2×1, no reshape


%% Sum own position
pos_sum = own_pos;

%% Add each neighbour position explicitly
for j = 1:N_all-1
    pos_sum = pos_sum + [x_hat_neighbors(1,j); x_hat_neighbors(2,j)];
end

%% Average over total count
x_c   = pos_sum / N_all;
end

== matlab function distributed_project_triangle_adjusted/MATLAB Function14 ==
  data: ID_i input; delta_i output double; N input; formation input
function delta_i = formation_calculator(ID_i, N, formation)
    %#codegen
    
    delta_i = [0; 0];
    
    if N <= 0 || ID_i < 1 || ID_i > N || N == 1
        return;
    end
    spacing = 0.5;
    switch formation
        case 1  % LINE (N ≤ 2)
            center = (N - 1) / 2;
            delta_i = double([(ID_i - 1 - center) * spacing; 0]);
            
        case 2  % CIRCLE (N ≥ 5)
            radius = spacing * N / (2 * pi);
            theta = 2 * pi * (ID_i - 1) / N;
            delta_i = radius * [cos(double(theta)); sin(double(theta))];
            
        case 3  % SQUARE (N = 4)
            half = spacing / 2;
            corners = [ half, -half, -half,  half;   % x-coordinates
                       -half, -half,  half,  half];  % y-coordinates
            delta_i = corners(:, ID_i);
            
        case 4  % TRIANGLE (N = 3)
            side = spacing * 2;
            h = sqrt(3) / 2 * side;
            vertices = [0,   -side/2,  side/2;    % x-coordinates
                       2*h/3, -h/3,   -h/3];     % y-coordinates
            delta_i = vertices(:, ID_i);
            
        otherwise
            delta_i = [0; 0];
    end
end

== matlab function distributed_project_triangle_adjusted/MATLAB Function15 ==
  data: N_final input; formation output
function formation = formation_selector(N_final)


    if N_final <= 0
        formation = 0;  % Invalid
        warning('Invalid number of agents: %d', N_final);
        return;
    end

    if N_final <= 2
        formation = 1;
    elseif N_final == 3
        formation = 4;
    elseif N_final == 4
        formation = 3;
    else
        formation = 2;
    end

end

== matlab function distributed_project_triangle_adjusted/MATLAB Function17 ==
  data: x_fused input; ei_pos_f output; x_c input; delta_i input; ei_norm output; x_c_raw input
function [ei_pos_f, ei_norm] = formation_error_calculator(...
                               x_fused, x_c, delta_i, x_c_raw)
%#codegen
persistent ei_prev;
if isempty(ei_prev)
    ei_prev = zeros(2,1);
end
ei_pos_raw = (x_c + delta_i) - x_fused(1:2);

%% Low-pass filter — smooth noise
alpha    = 0.167;   % Ts=0.01, tau=0.05s
ei_pos_f = (1-alpha)*ei_prev + alpha*ei_pos_raw;

%% Use raw norm for threshold (not filtered)
ei_norm = norm((x_c_raw + delta_i) - x_fused(1:2));
ei_prev = ei_pos_f;
end

== matlab function distributed_project_triangle_adjusted/MATLAB Function18 ==
  data: ei_pos input; ei_vel input; kp input; kd input; L input; vL output size=1; vR output size=1; theta input; w_scaled output; u output
function [vL, vR, w_scaled, u] = control_law(ei_pos, ei_vel, kp, kd, L, theta)
%#codegen

u = [0.0; 0.0];
w_scaled = double(0);
vL = double(0);
vR = double(0);

%% Deadband for spacing=0.3m
e_dead = 0.08;
if norm(ei_pos) < e_dead
    return;
end

u = kp * ei_pos - kd * ei_vel;

%% Tighter saturation for small formation
u_max  = 0.4;
u_norm = sqrt(u(1)^2 + u(2)^2);
if u_norm > u_max
    u = u * (u_max / u_norm);
end

v_lin =  cos(theta)*u(1) + sin(theta)*u(2);
w     = -sin(theta)*u(1) + cos(theta)*u(2);

w_scaled = w / (L/2);

v_max = 0.4;     % slower for small formation
w_max = 0.4;
v_lin    = max(-v_max, min(v_max, v_lin));
w_scaled = max(-w_max, min(w_max, w_scaled));

vL = v_lin - (L/2)*w_scaled;
vR = v_lin + (L/2)*w_scaled;
end

== matlab function distributed_project_triangle_adjusted/MATLAB Function8 ==
  data: ID_i input int32; msg output Bus: msgBus; x_i input; P_i input; t_now input
function msg = create_msg(ID_i, x_i, P_i, t_now)
%#codegen

% Create bus-compatible struct

msg = struct( ...
    'ID', int32(0), ...
    'x',  zeros(size(x_i)), ...
    'P',  zeros(size(P_i)), ...
    't',  0);

% Assign values
msg.ID = ID_i;
msg.x  = x_i;
msg.P  = P_i;
msg.t  = t_now;

end

== matlab function distributed_project_triangle_adjusted/MATLAB Function9 ==
  data: msg_in input; x_hat_neighbors output; neighbor_idx output; P_j_neighbours output; N output; my_id input; t_now input size=1
function [x_hat_neighbors, neighbor_idx, P_j_neighbours, N] = ...
         receive_msg(msg_in, my_id, t_now)
%#codegen

%% Fixed dimensions — must be constants for codegen
MAX_AGENTS  = 7;
STATE_DIM   = 3;
P_DIM       = 3;
T_WINDOW    = 5.0;   % seconds — max message age

N = 0;

for i = 1:length(msg_in)
    if msg_in(i).ID ~= 0   % assume ID=0 means empty slot
        N = N + 1;
    end
end


%% Fixed-size outputs — codegen requires known dimensions
x_hat_neighbors = zeros(STATE_DIM, MAX_AGENTS);
P_j_neighbours  = zeros(P_DIM, P_DIM, MAX_AGENTS);
neighbor_idx    = zeros(1, MAX_AGENTS);
N_neighbors     = 0;




%% Persistent store — holds latest message per agent slot
%% Indexed by agent ID (1..MAX_AGENTS)
persistent latest_x latest_P latest_t latest_valid

if isempty(latest_x)
    latest_x     = zeros(STATE_DIM, MAX_AGENTS);
    latest_P     = zeros(P_DIM, P_DIM, MAX_AGENTS);
    latest_t     = -inf(1, MAX_AGENTS);   % never received
    latest_valid = zeros(1, MAX_AGENTS);  % 0 = no data
end

%% ── Step 1: Update persistent store with incoming messages ────────
for k = 1:length(msg_in)
    id = msg_in(k).ID;

    %% Skip invalid IDs
    if id < 1 || id > N
        continue;
    end

    %% Skip own messages
    if id == my_id
        continue;
    end

    %% Keep only the latest message per ID
    if msg_in(k).t > latest_t(id)
        latest_x(:, id)      = msg_in(k).x;
        latest_P(:, :, id)   = msg_in(k).P;
        latest_t(id)         = msg_in(k).t;
        latest_valid(id)     = 1;
    end
end

%% ── Step 2: Collect valid neighbours within time window ───────────
for id = 1:N

    %% Skip self
    if id == my_id
        continue;
    end

    %% Skip slots never received
    if latest_valid(id) == 0
        continue;
    end

    %% Skip stale messages
    msg_age = t_now - latest_t(id);
    if msg_age > T_WINDOW || msg_age < 0
        continue;
    end

    %% Valid neighbour — add to output
    N_neighbors = N_neighbors + 1;
    x_hat_neighbors(:, N_neighbors) = latest_x(:, id);
    P_j_neighbours(:,:, N_neighbors) = latest_P(:,:, id);
    neighbor_idx(N_neighbors) = id;
end





end

== matlab function distributed_project_triangle_adjusted/Subsystem3/MATLAB Function1 ==
  data: pos_x input; x_next output; pos_y input; theta input; v input; a input; w input; P_next output; gyro_bias input
function [x_next, P_next] = local_ekf_predict(pos_x,pos_y, theta, v, a, w, gyro_bias)
% MOTION_UPDATE: Predicts the next state and covariance for a 2D vehicle
%
% Inputs:
%   x  - current state [x; y; theta; v]
%   P  - current state covariance (4x4)
%   u  - control input [a; omega] (acceleration, angular rate)
%   Q  - process noise covariance (4x4)
%   dt - time step Δt
%
% Outputs:
%   x_next - predicted next state
%   P_next - predicted next covariance

dt = 0.01;
%% In PreLoadFcn or MATLAB workspace:

sigma_x     = 0.01;
sigma_y     = 0.01;
sigma_theta = 0.005;

Q = diag([sigma_x^2*dt;
            sigma_y^2*dt;
                sigma_theta^2*dt]);
% Make P persistent across calls
persistent P;
    if isempty(P)
        P = eye(3) * 0.1;  % initialize first time
    end

% State prediction (nonlinear)
x_next = zeros(3,1);

              % angular velocity (yaw)
bias_z = gyro_bias(3);      % gyro bias (yaw)
v = norm(v);
a = norm(a);
x_next(1) = pos_x + v * cos(theta) * dt;
x_next(2) = pos_y + v * sin(theta) * dt;
x_next(3) = theta + w * dt;
%x_next(4) = v + a * dt;
%x_next(5) = bias_z;

% Jacobian F_k = ∂f/∂x
A = [ 1, 0, -v*sin(theta)*dt;
      0, 1,  v*cos(theta)*dt;
      0, 0,               1];               


% Covariance prediction
P_next = A * P * A' + Q;
P = P_next;
end

== matlab function distributed_project_triangle_adjusted/Subsystem3/MATLAB Function2 ==
  data: x_bar input; x_hat output; P_bar input; z_actual input; R input; H input; P_hat output; z_pred output
function [x_hat, P_hat, z_pred] = local_ekf_update(x_bar, P_bar, z_actual, R, H)
% EKF_UPDATE: Performs the measurement update step of an EKF
%
% Inputs:
%   x_bar - predicted state (from motion model)
%   P_bar - predicted covariance (from motion model)
%   z     - measurement vector
%   R     - measurement noise covariance
%   h     - function handle for measurement model h(x)
%   H_    - Jacobian H = dh/dx at x_bar
%
% Outputs:
%   x_hat - updated state estimate
%   P_hat - updated covariance estimate

% 1. Compute predicted measurement
% Measurement function evaluated at x
h = [ ...
    x_bar(1);  % gps_x
    x_bar(2);  % gps_y
    x_bar(3)   % theta
];

% Jacobian
z_pred = h;

% 2. Innovation
y = z_actual - z_pred;

% 4. Innovation covariance
S = H * P_bar * H' + R;
% Check condition number and add regularization if needed
    if rcond(S) < 1e-12
        % Add small diagonal perturbation
        S = S + 1e-6 * eye(size(S));
        warning('S matrix near singular, added regularization');
    end
% 5. Kalman gain
W = (P_bar * H') * pinv(S);

% 6. Update state
x_hat = x_bar + W * y;

% 7. Update covariance
I = eye(length(x_bar));
P_hat = (I - W * H) * P_bar;

end

== matlab function distributed_project_triangle_adjusted/Subsystem3/MATLAB Function3 ==
  data: z input; R output
function R = getR(z)
    % Compute measurement noise covariance matrix
    % z: matrix where rows = samples, columns = different sensors
    % Returns: full covariance matrix (including cross-terms)
    
    z_detrended = z - mean(z, 1);  % Remove mean from each column
    R = cov(z_detrended);           % Full covariance matrix
    
end

== matlab function distributed_project_triangle_adjusted/Subsystem3/MATLAB Function4 ==
  data: H output; x_ input size=[3 1]
function H = compute_jacobian(x_)
assert(numel(x_) == 3);
% Ensure column vector
x_ = x_(:);



% Measurement function evaluated at x
h = [ ...
    x_(1);  % gps_x
    x_(2);  % gps_y
    x_(3)  % imu_theta
  % gyro_bias
];

% Jacobian
H = eye(3);

end

== matlab function distributed_project_triangle_adjusted/Subsystem3/MATLAB Function5 ==
  data: gps_x input; z_actual output; gps_y input; theta_imu input; v_enc input; w_imu input
function z_actual = get_z(gps_x, gps_y, theta_imu, v_enc, w_imu)
v_enc = norm(v_enc);
z_actual = [gps_x; gps_y; theta_imu];

== matlab function distributed_project_triangle_adjusted/Subsystem4/MATLAB Function ==
  data: vR input; vL input; fx output; fy output; vx_actual input; vy_actual input; theta input; w_desired input; tau_z output; w_actual input
function [fx, fy, tau_z] = planar_control(vR, vL, vx_actual, vy_actual, theta, ...
                                  w_desired, w_actual)
%#codegen

% --- linear control (vector form) ---
Kp_pos = 10;

% desired velocity in world frame
v_desired = (vR + vL)/2;
vx_des = v_desired * cos(theta);
vy_des = v_desired * sin(theta);

% force based on velocity error
fx = Kp_pos * (vx_des - vx_actual);
fy = Kp_pos * (vy_des - vy_actual);
%#codegen
%% Simple P controller on angular velocity
%% tau = I * (w_desired - w_actual) / Ts
Kp_heading = 0.3;        % tune this
tau_z = Kp_heading * (w_desired - w_actual);
if vR==0 || vL==0
    tau_z = 0;
    fx = 0;
    fy = 0;
end
%% Torque must be 3x1 for Spherical Primitive (x,y,z torques)
%% Only Z torque for planar rotation
tau = [0; 0; tau_z];
end

== matlab function distributed_project_triangle_adjusted/MATLAB Function ==
  data: x output; lat input; y output; lon input
function [x,y] = getXY(lat, lon)

% Reference point
persistent lat0 lon0 initialized

if isempty(initialized)
    lat0 = lat;
    lon0 = lon;
    initialized = true;
end



% Convert to radians
lat0_rad = deg2rad(lat0);
lon0_rad = deg2rad(lon0);
lat_rad  = deg2rad(lat);
lon_rad  = deg2rad(lon);

% Earth radius
R = 6371000; % meters

% Compute local x, y
lat_avg = (lat_rad + lat0_rad)/2;
x = R * (lon_rad - lon0_rad) * cos(lat_avg); % east
y = R * (lat_rad - lat0_rad);                 % north

== matlab function distributed_project_triangle_adjusted/MATLAB Function16 ==
  data: ID_i input int32; msg output Bus: msgBus; x_i input; P_i input; t_now input
function msg = create_msg(ID_i, x_i, P_i, t_now)
%#codegen

% Create bus-compatible struct

msg = struct( ...
    'ID', int32(0), ...
    'x',  zeros(size(x_i)), ...
    'P',  zeros(size(P_i)), ...
    't',  0);

% Assign values
msg.ID = ID_i;
msg.x  = x_i;
msg.P  = P_i;
msg.t  = t_now;

end

== matlab function distributed_project_triangle_adjusted/Subsystem4/MATLAB Function1 ==
  data: vL_actual input; v_xyz output; vR_actual input; theta input
function v_xyz = compute_velocity(vL_actual, vR_actual, theta)
%#codegen

v_true = (vL_actual + vR_actual) / 2;
vx = v_true * cos(theta);
vy = v_true * sin(theta);
vz = 0;

v_xyz = [vx; vy; vz];   % 3x1 vector

end

== matlab function distributed_project_triangle_adjusted/Subsystem4/MATLAB Function2 ==
  data: vL_actual input; w_true output; vR_actual input; L input
function w_true = compute_angular_velocity(vL_actual, vR_actual, L)
%#codegen

w_true = (vR_actual - vL_actual) / L;

end

== matlab function distributed_project_triangle_adjusted/Subsystem4/MATLAB Function24 ==
  data: quat input; theta output
function theta = quat_to_angle(quat)
%#codegen

% normalize (important if coming from simulation)
quat = quat / norm(quat);

w = quat(1);
z = quat(4);

theta = 2 * atan2(z, w);

end
